simulink library "INT_TIntkVUs_VD"  (R2016b)
settings: Solver=VariableStepAuto  StartTime=0.0  StopTime=10.0  RelTol=1e-3
settings Model: Creator=zhoutinglin  LastModifiedBy=zhoutinglin

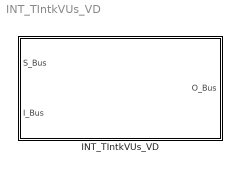
== system INT_TIntkVUs_VD ==
  INT_TIntkVUs_VD : Subsystem

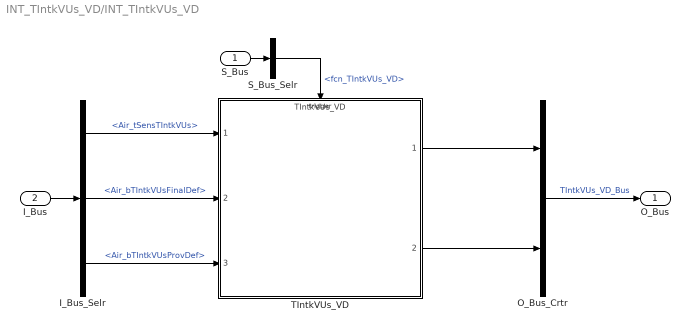
== system INT_TIntkVUs_VD/INT_TIntkVUs_VD ==
  S_Bus : Inport
  I_Bus : Inport  Port=2
  I_Bus_Selr : BusSelector  OutputSignals=Air_tSensTIntkVUs,Air_bTIntkVUsFinalDef,Air_bTIntkVUsProvDef
  O_Bus_Crtr : BusCreator  Inputs=2
  S_Bus_Selr : BusSelector  OutputSignals=fcn_TIntkVUs_VD
  TIntkVUs_VD : ModelReference  ModelNameDialog=TIntkVUs_VD  SimulationMode=Normal  ModelReferenceVersion=1.16  TriggerPortName=function  TriggerPortTriggerType=function-call  TriggerPortStatesWhenEnabling=held
  O_Bus : Outport
  wires:
  S_Bus_Selr/1 -> TIntkVUs_VD/Trigger  "<fcn_TIntkVUs_VD>"
  S_Bus/1 -> S_Bus_Selr/1
  I_Bus/1 -> I_Bus_Selr/1
  I_Bus_Selr/1 -> TIntkVUs_VD/1  "<Air_tSensTIntkVUs>"
  I_Bus_Selr/2 -> TIntkVUs_VD/2  "<Air_bTIntkVUsFinalDef>"
  I_Bus_Selr/3 -> TIntkVUs_VD/3  "<Air_bTIntkVUsProvDef>"
  O_Bus_Crtr/1 -> O_Bus/1  "TIntkVUs_VD_Bus"
  TIntkVUs_VD/1 -> O_Bus_Crtr/1
  TIntkVUs_VD/2 -> O_Bus_Crtr/2
